simulink model "slider_button_demo"  (Simulink 7.3)
settings: Solver=ode45  StartTime=0.0  StopTime=inf  RelTol=1e-3
libraries: simulink x5, waijung_addon_module x1
settings Model: Creator=Krisada  LastModifiedBy=Krisada

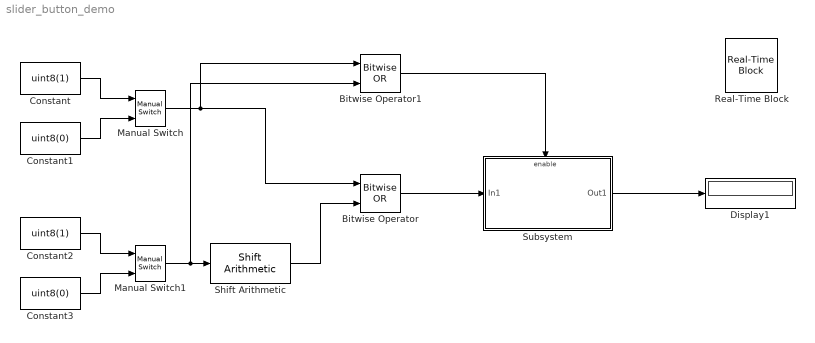
== system slider_button_demo ==
  Bitwise Operator : simulink/Logic and Bit Operations/Bitwise Operator  logicop=OR  UseBitMask=off  NumInputPorts=2  BitMask=bin2dec('00000011')  BitMaskRealWorld=Stored Integer
  Bitwise Operator1 : simulink/Logic and Bit Operations/Bitwise Operator  logicop=OR  UseBitMask=off  NumInputPorts=2  BitMask=bin2dec('00000011')  BitMaskRealWorld=Stored Integer
  Constant : Constant  Value=uint8(1)  OutDataType=fixdt(1, 16)  OutScaling=2^0  SampleTime=.1
  Constant1 : Constant  Value=uint8(0)  OutDataType=fixdt(1, 16)  OutScaling=2^0  SampleTime=.1
  Constant2 : Constant  Value=uint8(1)  OutDataType=fixdt(1, 16)  OutScaling=2^0  SampleTime=.1
  Constant3 : Constant  Value=uint8(0)  OutDataType=fixdt(1, 16)  OutScaling=2^0  SampleTime=.1
  Display1 : Display
  Manual Switch : simulink/Signal Routing/Manual Switch  SystemSampleTime=-1  sw=0  action=0  varsize=off
  Manual Switch1 : simulink/Signal Routing/Manual Switch  SystemSampleTime=-1  sw=0  action=0  varsize=off
  Real-Time Block : waijung_addon_module/Real-Time Block  Priority=0  setting=Default  sampletime=-1
  Shift Arithmetic : simulink/Logic and Bit Operations/Shift Arithmetic  SystemSampleTime=-1  nBitShiftRight=-1  nBinPtShiftRight=0
  Subsystem : Subsystem
  wires:
  Constant/1 -> Manual Switch/1
  Constant1/1 -> Manual Switch/2
  Constant2/1 -> Manual Switch1/1
  Constant3/1 -> Manual Switch1/2
  Manual Switch1/1 -> Shift Arithmetic/1, Bitwise Operator1/2
  Manual Switch/1 -> Bitwise Operator/1, Bitwise Operator1/1
  Shift Arithmetic/1 -> Bitwise Operator/2
  Subsystem/1(Out1) -> Display1/1
  Bitwise Operator/1 -> Subsystem/1(In1)
  Bitwise Operator1/1 -> Subsystem/Enable

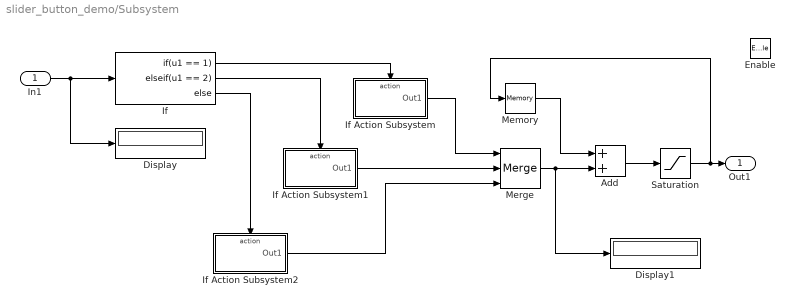
== system slider_button_demo/Subsystem ==
  In1 : Inport
  Enable : EnablePort
  Add : Sum  OutDataType=fixdt(1, 16)  OutScaling=2^-10
  Display : Display
  Display1 : Display
  If : If  IfExpression=u1 == 1  ElseIfExpressions=u1 == 2
  If Action Subsystem : Subsystem  TreatAsAtomicUnit=on
  If Action Subsystem1 : Subsystem  TreatAsAtomicUnit=on
  If Action Subsystem2 : Subsystem  TreatAsAtomicUnit=on
  Memory : Memory  InheritSampleTime=on
  Merge : Merge  Inputs=3
  Saturation : Saturate  UpperLimit=13  LowerLimit=-13  OutDataType=fixdt(1, 16)  OutScaling=2^0
  Out1 : Outport
  wires:
  In1/1 -> If/1, Display/1
  If/1 -> If Action Subsystem/Action
  If/2 -> If Action Subsystem1/Action
  If/3 -> If Action Subsystem2/Action
  If Action Subsystem/1(Out1) -> Merge/1
  If Action Subsystem1/1(Out1) -> Merge/2
  If Action Subsystem2/1(Out1) -> Merge/3
  Memory/1 -> Add/1
  Merge/1 -> Add/2, Display1/1
  Add/1 -> Saturation/1
  Saturation/1 -> Out1/1, Memory/1

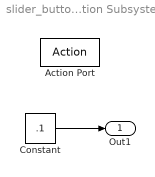
== system slider_button_demo/Subsystem/If Action Subsystem ==
  Action Port : ActionPort  ActionType=then
  Constant : Constant  Value=.1  OutDataType=fixdt(1, 16)  OutScaling=2^0
  Out1 : Outport  OutDataType=fixdt(1, 16)  OutScaling=2^0
  wires:
  Constant/1 -> Out1/1

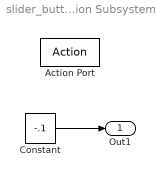
== system slider_button_demo/Subsystem/If Action Subsystem1 ==
  Action Port : ActionPort  ActionType=elseif
  Constant : Constant  Value=-.1  OutDataType=fixdt(1, 16)  OutScaling=2^0
  Out1 : Outport  OutDataType=fixdt(1, 16)  OutScaling=2^0
  wires:
  Constant/1 -> Out1/1

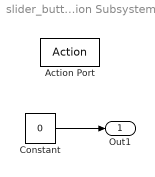
== system slider_button_demo/Subsystem/If Action Subsystem2 ==
  Action Port : ActionPort  ActionType=else
  Constant : Constant  Value=0  OutDataType=fixdt(1, 16)  OutScaling=2^0
  Out1 : Outport  OutDataType=fixdt(1, 16)  OutScaling=2^0
  wires:
  Constant/1 -> Out1/1
